simulink model "QuaterSuspension"  (R2017a)
settings: Solver=VariableStepAuto  StartTime=0.0  StopTime=10  FixedStep=0.01  RelTol=1e-3
libraries: simulink x1
settings Model: Creator=uidm1296  LastModifiedBy=uidm1296

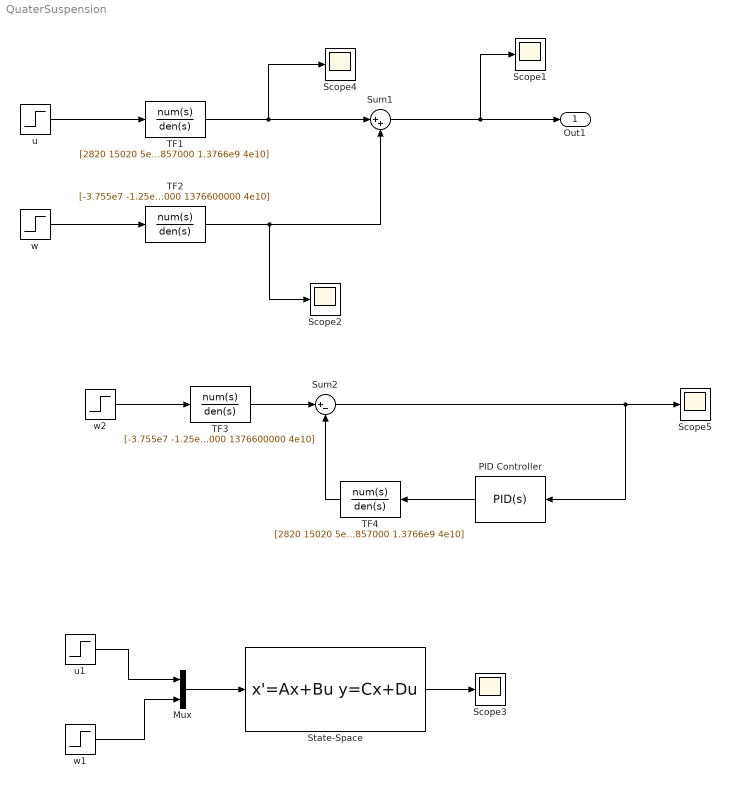
== system QuaterSuspension ==
  Mux : Mux  Inputs=2
  PID Controller : simulink/Continuous/PID Controller  Controller=PID  TimeDomain=Continuous-time  SampleTime=-1  IntegratorMethod=Forward Euler  FilterMethod=Forward Euler  Form=Parallel  UseFilter=on  ControllerParametersSource=internal  P=4.5e5  I=2e4  D=8.1e5  N=100  InitialConditionSource=internal  InitialConditionForIntegrator=0  InitialConditionForFilter=0  ExternalReset=none  LimitOutput=off  UpperSaturationLimit=inf  LowerSaturationLimit=-inf  LinearizeAsGain=on  AntiWindupMode=none  Kb=1  TrackingMode=off  Kt=1  PParamMin=[]  PParamMax=[]  IParamMin=[]  IParamMax=[]  DParamMin=[]  DParamMax=[]  NParamMin=[]  NParamMax=[]  KbParamMin=[]  KbParamMax=[]  KtParamMin=[]  KtParamMax=[]  POutMin=[]  POutMax=[]  IOutMin=[]  IOutMax=[]  DOutMin=[]  DOutMax=[]  NOutMin=[]  NOutMax=[]  KbOutMin=[]  KbOutMax=[]  KtOutMin=[]  KtOutMax=[]  IntegratorOutMin=[]  IntegratorOutMax=[]  FilterOutMin=[]  FilterOutMax=[]  SumOutMin=[]  SumOutMax=[]  SumI1OutMin=[]  SumI1OutMax=[]  SumI2OutMin=[]  SumI2OutMax=[]  SumI3OutMin=[]  SumI3OutMax=[]  SumDOutMin=[]  SumDOutMax=[]  SaturationOutMin=[]  SaturationOutMax=[]  IntegratorContinuousStateAttributes=''  IntegratorStateMustResolveToSignalObject=off  IntegratorRTWStateStorageClass=Auto  FilterContinuousStateAttributes=''  FilterStateMustResolveToSignalObject=off  FilterRTWStateStorageClass=Auto  DifferentiatorICPrevScaledInput=0  DifferentiatorOutMin=[]  DifferentiatorOutMax=[]  InitialConditionSetting=State (most efficient)
  Scope{1..5} (5 alike) : Scope
  State-Space : StateSpace  A=[0 -32 0 250; 1 -0.14 0 1.09375; 0 0 0 -1562.5; 0 0 1 -46.9375]  B=[1 0; 0 0; 0 500000; 0 15020]  C=[0 0.0004 0 -0.00313]  D=[0 0]  X0=0
  Sum1 : Sum  Inputs=|++
  Sum2 : Sum  Inputs=|+-
  TF1 : TransferFcn  Numerator=[2820 15020 5e5]  Denominator=[8e5 38537000 1480857000 1.3766e9 4e10]
  TF2 : TransferFcn  Numerator=[-3.755e7 -1.25e9 0 0]  Denominator=[8e5 38537000 1480857000 1376600000 4e10]
  TF3 : TransferFcn  Numerator=[-3.755e7 -1.25e9 0 0]  Denominator=[8e5 38537000 1480857000 1376600000 4e10]
  TF4 : TransferFcn  Numerator=[2820 15020 5e5]  Denominator=[8e5 38537000 1480857000 1.3766e9 4e10]
  u : Step  After=0  SampleTime=0
  u1 : Step  After=0  SampleTime=0
  w : Step  After=0.1  SampleTime=0
  w1 : Step  After=0.1  SampleTime=0
  w2 : Step  After=0.1  SampleTime=0
  Out1 : Outport
  wires:
  u/1 -> TF1/1
  w/1 -> TF2/1
  TF2/1 -> Sum1/2, Scope2/1
  TF1/1 -> Sum1/1, Scope4/1
  Sum1/1 -> Scope1/1, Out1/1
  u1/1 -> Mux/1
  w1/1 -> Mux/2
  Mux/1 -> State-Space/1
  State-Space/1 -> Scope3/1
  w2/1 -> TF3/1
  TF3/1 -> Sum2/1
  PID Controller/1 -> TF4/1
  Sum2/1 -> Scope5/1, PID Controller/1
  TF4/1 -> Sum2/2
